simulink model "MPG_MG_PLL_orig"  (R2021b)
settings: Solver=VariableStepAuto  StartTime=0.0  StopTime=1  RelTol=1e-3
model workspace (MAT data in the model file):
  Ts = Simulink.Parameter
  Ts.Value = 5e-06
  Ts.DataType = 'auto'
  Ts.Complexity = 'real'
  Ts.Dimensions = [1 1]
  secondary_on = Simulink.Parameter
  secondary_on.DataType = 'auto'
  secondary_on.Complexity = 'real'
  secondary_on.Dimensions = [0 0]
values from neighbouring files (symbols this model uses):
  A = zeros(4,4)    [MPC_MG_script_raw_dmpc.m]    (also in MPG_MG_July.m = [0 1 1 1; 1 0 0 0; 1 0 0 0; 1 0 0 0]; MPG_MG_freq_script.m = ones(4) - eye(4); Script.m = [0 1 1 1 ; 1 0 1 1 ; 1 1 0 1 ; 1 1 1 0])
  C_f = 50e-6    (= 5e-05)    [Four_DG_MG_PrimaryOnlyScript.m]    (also in MPC_MG_script.m; MPC_MG_script_raw_dmpc.m; MPC_MG_secondary_script.m; MPG_MG_July.m)
  f_c = 5000    [Four_DG_MG_PrimaryOnlyScript.m]    (also in MPC_MG_script.m = 40000; MPC_MG_script_raw_dmpc.m = 40000; MPC_MG_secondary_script.m = 40000; MPG_MG_July.m = 50000)
  kL = 1e-5    (= 1e-05)    [Four_DG_MG_PrimaryOnlyScript.m]    (also in MPC_MG_script.m = 1e-08; MPC_MG_script_raw_dmpc.m = 1e-08; MPC_MG_secondary_script.m = 1e-07; MPG_MG_July.m = 1e-07)
  L_f = 1.35e-3    (= 0.00135)    [Four_DG_MG_PrimaryOnlyScript.m]    (also in MPC_MG_script.m; MPC_MG_script_raw_dmpc.m; MPC_MG_secondary_script.m; MPG_MG_July.m)
  L_in1 = 0.35e-3    (= 0.00035)    [Four_DG_MG_PrimaryOnlyScript.m]    (also in MPC_MG_script.m; MPC_MG_script_raw_dmpc.m; MPC_MG_secondary_script.m; MPG_MG_July.m)
  L_in2 = 0.35e-3    (= 0.00035)    [Four_DG_MG_PrimaryOnlyScript.m]    (also in MPC_MG_script.m; MPC_MG_script_raw_dmpc.m; MPC_MG_secondary_script.m; MPG_MG_July.m)
  L_in4 = 0.35e-3    (= 0.00035)    [Four_DG_MG_PrimaryOnlyScript.m]    (also in MPC_MG_script.m; MPC_MG_script_raw_dmpc.m; MPC_MG_secondary_script.m; MPG_MG_July.m)
  lambda1 = [30000 50000 90000 50000]'    [MPC_MG_script_raw_dmpc.m]    (also in MPG_MG_July.m = [4 4 4 4]'; MPG_MG_freq_script.m = [3 3 3 3]'; Script.m = [1 1 1 1]')
  lambda2 = [5 6 7 6]'    [MPC_MG_script_raw_dmpc.m]    (also in MPG_MG_July.m = [0.5e-2 0.5e-2 0.5e-2 0.5e-2]'; MPG_MG_freq_script.m = [1.1 1.9 1.5 1.2]'; Script.m = [0.8e-2 0.8e-2 0.8e-2 0.8e-2]')
  lambda3 = [80000 80000 900000 80000]'    [MPC_MG_script_raw_dmpc.m]    (also in MPG_MG_July.m = [1e-3 1e-3 1e-3 1e-3]'; MPG_MG_freq_script.m = [9e-4 1.2e-2 3e-3 3e-3]'; Script.m = [1.5e-3 1.5e-3 1.5e-3 1.5e-3]')
  LD_ref1 = 800e-6    (= 0.0008)    [Four_DG_MG_PrimaryOnlyScript.m]    (also in MPC_MG_script.m = 0.0003; MPC_MG_script_raw_dmpc.m = 0.0003; MPC_MG_secondary_script.m = 0.0001; MPG_MG_July.m = 0.0004)
  lo_co = 0.2    [Four_DG_MG_PrimaryOnlyScript.m]    (also in MPC_MG_script.m = 0.05; MPC_MG_script_raw_dmpc.m; MPC_MG_secondary_script.m = 0.08; MPG_MG_July.m = 0.15)
  m_p1 = 9.4e-5/droopDivide    (= 9.4e-05)    [Four_DG_MG_PrimaryOnlyScript.m]    (also in MPC_MG_script.m; MPC_MG_script_raw_dmpc.m; MPC_MG_secondary_script.m; MPG_MG_July.m)
  m_p2 = 9.4e-5/droopDivide    (= 9.4e-05)    [Four_DG_MG_PrimaryOnlyScript.m]    (also in MPC_MG_script.m; MPC_MG_script_raw_dmpc.m; MPC_MG_secondary_script.m; MPG_MG_July.m)
  m_p3 = 12.5e-5/droopDivide    (= 0.000125)    [Four_DG_MG_PrimaryOnlyScript.m]    (also in MPC_MG_script.m; MPC_MG_script_raw_dmpc.m; MPC_MG_secondary_script.m; MPG_MG_July.m)
  m_p4 = 12.5e-5/droopDivide    (= 0.000125)    [Four_DG_MG_PrimaryOnlyScript.m]    (also in MPC_MG_script.m; MPC_MG_script_raw_dmpc.m; MPC_MG_secondary_script.m; MPG_MG_July.m)
  N = 3    [MPG_MG_July.m]    (also in MPG_MG_freq_script.m = 2; Script.m = 5)
  n_q1 = 1.3e-3/droopDivide2    (= 0.00013)    [Four_DG_MG_PrimaryOnlyScript.m]    (also in MPC_MG_script.m; MPC_MG_script_raw_dmpc.m; MPC_MG_secondary_script.m; MPG_MG_July.m)
  n_q2 = 1.3e-3/droopDivide2    (= 0.00013)    [Four_DG_MG_PrimaryOnlyScript.m]    (also in MPC_MG_script.m; MPC_MG_script_raw_dmpc.m; MPC_MG_secondary_script.m; MPG_MG_July.m)
  n_q4 = 1.5e-3/droopDivide2    (= 0.00015)    [Four_DG_MG_PrimaryOnlyScript.m]    (also in MPC_MG_script.m; MPC_MG_script_raw_dmpc.m; MPC_MG_secondary_script.m; MPG_MG_July.m)
  Pmax = [45e3 45e3 37e3 37e3]'    [MPG_MG_July.m]    (also in MPG_MG_freq_script.m; Script.m)
  R_f = 0.1    [Four_DG_MG_PrimaryOnlyScript.m]    (also in MPC_MG_script.m; MPC_MG_script_raw_dmpc.m; MPC_MG_secondary_script.m; MPG_MG_July.m)
  R_in1 = 0.03    [Four_DG_MG_PrimaryOnlyScript.m]    (also in MPC_MG_script.m; MPC_MG_script_raw_dmpc.m; MPC_MG_secondary_script.m; MPG_MG_July.m)
  R_in2 = 0.03    [Four_DG_MG_PrimaryOnlyScript.m]    (also in MPC_MG_script.m; MPC_MG_script_raw_dmpc.m; MPC_MG_secondary_script.m; MPG_MG_July.m)
  R_in4 = 0.03    [Four_DG_MG_PrimaryOnlyScript.m]    (also in MPC_MG_script.m; MPC_MG_script_raw_dmpc.m; MPC_MG_secondary_script.m; MPG_MG_July.m)
  time_thresh = 0.6    [Four_DG_MG_PrimaryOnlyScript.m]    (also in MPC_MG_script_raw_dmpc.m = 1.5; MPC_MG_secondary_script.m = 2; MPG_MG_July.m = 0.5; MPG_MG_freq_script.m = 0.5)
  Ts = 10e-6    (= 1e-05)    [Four_DG_MG_PrimaryOnlyScript.m]    (also in MPC_MG_script.m; MPC_MG_script_raw_dmpc.m; MPC_MG_secondary_script.m; MPG_MG_July.m)
  Tsamp = 0.1    [MPG_MG_July.m]    (also in MPG_MG_freq_script.m; Script.m)
  V_nom = 220*sqrt(2)    [Four_DG_MG_PrimaryOnlyScript.m]    (also in MPC_MG_script.m; MPC_MG_script_raw_dmpc.m; MPC_MG_secondary_script.m; MPG_MG_July.m)
  Vdc = 600    [Four_DG_MG_PrimaryOnlyScript.m]    (also in MPC_MG_script.m; MPC_MG_script_raw_dmpc.m; MPC_MG_secondary_script.m; MPG_MG_July.m)
  w_c_high = 2*pi*50    (= 314.159265359)    [Four_DG_MG_PrimaryOnlyScript.m]    (also in MPC_MG_script.m; MPC_MG_script_raw_dmpc.m; MPC_MG_secondary_script.m; MPG_MG_July.m)
  w_nom = 2*pi*50    (= 314.159265359)    [Four_DG_MG_PrimaryOnlyScript.m]    (also in MPC_MG_script.m; MPC_MG_script_raw_dmpc.m; MPC_MG_secondary_script.m; MPG_MG_July.m)
undefined symbols (not defined in the file or in its folder): i
libraries: spsThreePhaseSeriesRLCBranchLib x18, spsabctodq0Lib x16, spsThreePhaseVIMeasurementLib x15, eeGeneralControl x15, dspswit3 x5, spsDCVoltageSourceLib x5, spsSeriesRLCBranchLib x5, spsTwoLevelConverterLib x5, slpidlib x5, spsAlphaBetaZerotodq0Lib x4, spsSecondOrderFilterLib x4, spsThreePhaseSeriesRLCLoadLib x2
(part 1 of 6)
settings Model: SimulationMode=accelerator  Creator=Linh  LastModifiedBy=Linh
settings SolverCC: AlgebraicLoopSolver=TrustRegion
settings DataIOCC: ReturnWorkspaceOutputs=off
settings DebuggingCC: SFMachineParentedDataDiag=warning

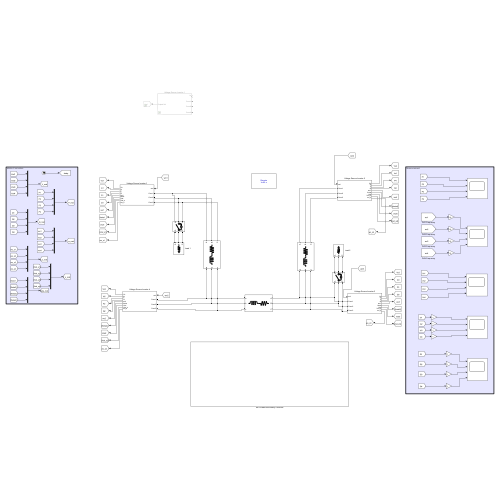
[thumbnail: Simulink's stored preview of the top-level diagram]
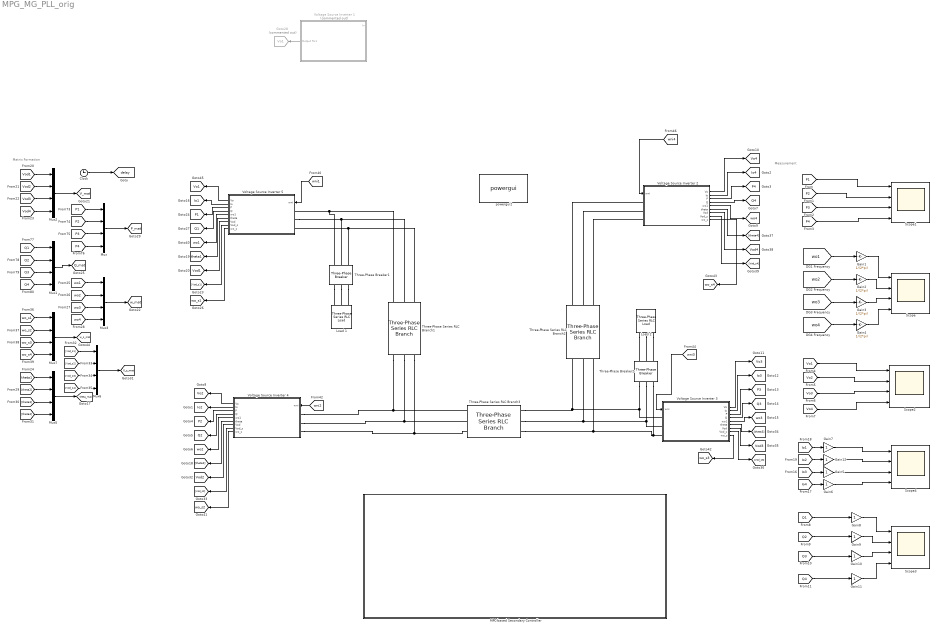
== system MPG_MG_PLL_orig ==
  note: Matrix Formation
  note: Measurement
  Clock : Clock
  Gain{1..4} (4 alike) : Gain  Gain=1/(2*pi)
  Gain{5..12} (8 alike) : Gain
  Goto28 : Goto  Commented=on  GotoTag=Vo1  TagVisibility=global
  Load 1 : spsThreePhaseSeriesRLCLoadLib/Three-Phase Series RLC Load  LConnTagsString=A|B|C  Configuration=Y (grounded)  NominalVoltage=220*sqrt(3)  Vabc=[1e3 1e3 1e3]  Vabcp=[1e3 1e3 1e3]  NominalFrequency=50  UnbalancedPower=off  ActivePower=4.285e3  InductivePower=0  CapacitivePower=0  Pabc=[10e3 9e3 11e3]  QLabc=[100 90 110]  QCabc=[100 90 110]  Pabcp=[10e3 9e3 11e3]  QLabcp=[100 90 110]  QCabcp=[100 90 110]  Measurements=Branch voltages and currents  LoadType=constant Z
  Load 2 : spsThreePhaseSeriesRLCLoadLib/Three-Phase Series RLC Load  LConnTagsString=A|B|C  Configuration=Y (grounded)  NominalVoltage=220*sqrt(3)  Vabc=[1e3 1e3 1e3]  Vabcp=[1e3 1e3 1e3]  NominalFrequency=50  UnbalancedPower=off  ActivePower=2.045e3  InductivePower=0  CapacitivePower=0  Pabc=[10e3 9e3 11e3]  QLabc=[100 90 110]  QCabc=[100 90 110]  Pabcp=[10e3 9e3 11e3]  QLabcp=[100 90 110]  QCabcp=[100 90 110]  Measurements=Branch voltages and currents  LoadType=constant Z
  MPC-based Secondary Controller : Subsystem
  Mux{,1..3,5..7} (7 alike) : Mux
  Scope{,1..4} (5 alike) : Scope  NumInputPorts=4
  Three-Phase Series RLC Branch1 : spsThreePhaseSeriesRLCBranchLib/Three-Phase Series RLC Branch  LConnTagsString=A|B|C  RConnTagsString=A|B|C  BranchType=RL  Resistance=0.01  Inductance=2.5e-3  Capacitance=1e-6  Measurements=Branch voltages and currents
  Three-Phase Series RLC Branch2 : spsThreePhaseSeriesRLCBranchLib/Three-Phase Series RLC Branch  LConnTagsString=A|B|C  RConnTagsString=A|B|C  BranchType=RL  Resistance=0.01  Inductance=2.5e-3  Capacitance=1e-6  Measurements=Branch voltages and currents
  Three-Phase Series RLC Branch3 : spsThreePhaseSeriesRLCBranchLib/Three-Phase Series RLC Branch  LConnTagsString=A|B|C  RConnTagsString=A|B|C  BranchType=RL  Resistance=0.01  Inductance=2.5e-3  Capacitance=1e-6  Measurements=Branch voltages and currents
  Three-Phase Breaker1 : spsThreePhaseBreakerLib/Three-Phase Breaker  InitialState=open  SwitchA=on  SwitchB=on  SwitchC=on  SwitchTimes=[0 11]  External=off  BreakerResistance=0.01  SnubberResistance=1e6  SnubberCapacitance=inf  Measurements=None
  Three-Phase Breaker2 : spsThreePhaseBreakerLib/Three-Phase Breaker  InitialState=open  SwitchA=on  SwitchB=on  SwitchC=on  SwitchTimes=[0.75 11]  External=off  BreakerResistance=0.01  SnubberResistance=1e6  SnubberCapacitance=inf  Measurements=None
  Voltage Source Inverter 1 : Subsystem  Commented=on  mask{w_nom=w_nom, V_nom=V_nom, modT=1/f_c, m_p=m_p2, n_q=n_q2, LD_ref=LD_ref1, k_LD=kL, w_c_high=[1 w_c_high], R_f=R_f, L_f=L_f, C_f=C_f, R_in=R_in2, L_in=L_in2}
      mask prompts: w_nom "Nominal frequency (radian)"; V_nom "Nominal voltage"; modT "Sampling Time"; m_p "P-w gain"; n_q "Q-V gain"; LD_ref "Reference virtual impedance (H)"; k_LD "Virtual impedance Q gain"; w_c_high "High-pass filter denominator:"; R_f "Inductor resistance:"; L_f "Filter inductance"; C_f "Filter capacitance"; R_in "Resistance coupling"; L_in "Inductance coupling"
      mask TypeOptions w_nom: w_nom/Value
      mask TypeOptions V_nom: V_nom/Value
      mask TypeOptions modT:
      | Model Predictive Control
      | /Ts
      mask TypeOptions m_p: Droop for secondary control2/Gain5/Gain
      mask TypeOptions n_q: Droop for secondary control2/Gain4/Gain
      mask TypeOptions LD_ref: LD_ref/Value
      mask TypeOptions k_LD: k_LD/Gain
      mask TypeOptions w_c_high: High-Pass Filter/Denominator
      mask TypeOptions R_f:
      | Three-Phase
      | Series RLC Branch/Resistance
      mask TypeOptions L_f:
      | Three-Phase
      | Series RLC Branch/Inductance
      mask TypeOptions C_f:
      | Three-Phase
      | Series RLC Branch2/Capacitance
      mask TypeOptions R_in:
      | Three-Phase
      | Series RLC Branch1/Resistance
      mask TypeOptions L_in:
      | Three-Phase
      | Series RLC Branch1/Inductance
      mask DialogControl ParameterGroupVar Prompt: Microgrid-wide values
      mask DialogControl Container5 Prompt: Droop value
      mask DialogControl Container8 Prompt: Filter
  Voltage Source Inverter 2 : Subsystem  mask{w_nom=w_nom, V_nom=V_nom, modT=1/f_c, m_p=m_p4, n_q=n_q4, LD_ref=LD_ref1, k_LD=kL, w_c_high=[1 w_c_high], R_f=R_f, L_f=L_f, C_f=C_f, R_in=R_in4, L_in=L_in4}
      mask prompts: w_nom "Nominal frequency (radian)"; V_nom "Nominal voltage"; modT "Sampling Time"; m_p "P-w gain"; n_q "Q-V gain"; LD_ref "Reference virtual impedance (H)"; k_LD "Virtual impedance Q gain"; w_c_high "High-pass filter denominator:"; R_f "Inductor resistance:"; L_f "Filter inductance"; C_f "Filter capacitance"; R_in "Resistance coupling"; L_in "Inductance coupling"
      mask TypeOptions w_nom: w_nom/Value
      mask TypeOptions V_nom: V_nom/Value
      mask TypeOptions modT:
      | Model Predictive Control
      | /Ts
      mask TypeOptions m_p: Droop for secondary control2/Gain5/Gain
      mask TypeOptions n_q: Droop for secondary control2/Gain4/Gain
      mask TypeOptions LD_ref: LD_ref/Value
      mask TypeOptions k_LD: k_LD/Gain
      mask TypeOptions w_c_high: High-Pass Filter/Denominator
      mask TypeOptions R_f:
      | Three-Phase
      | Series RLC Branch/Resistance
      mask TypeOptions L_f:
      | Three-Phase
      | Series RLC Branch/Inductance
      mask TypeOptions C_f:
      | Three-Phase
      | Series RLC Branch2/Capacitance
      mask TypeOptions R_in:
      | Three-Phase
      | Series RLC Branch1/Resistance
      mask TypeOptions L_in:
      | Three-Phase
      | Series RLC Branch1/Inductance
      mask DialogControl ParameterGroupVar Prompt: Microgrid-wide values
      mask DialogControl Container5 Prompt: Droop value
      mask DialogControl Container8 Prompt: Filter
  Voltage Source Inverter 3 : Subsystem  mask{w_nom=w_nom, V_nom=V_nom, modT=1/f_c, m_p=m_p4, n_q=n_q4, LD_ref=LD_ref1, k_LD=kL, w_c_high=[1 w_c_high], R_f=R_f, L_f=L_f, C_f=C_f, R_in=R_in4, L_in=L_in4}
      mask prompts: w_nom "Nominal frequency (radian)"; V_nom "Nominal voltage"; modT "Sampling Time"; m_p "P-w gain"; n_q "Q-V gain"; LD_ref "Reference virtual impedance (H)"; k_LD "Virtual impedance Q gain"; w_c_high "High-pass filter denominator:"; R_f "Inductor resistance:"; L_f "Filter inductance"; C_f "Filter capacitance"; R_in "Resistance coupling"; L_in "Inductance coupling"
      mask TypeOptions w_nom: w_nom/Value
      mask TypeOptions V_nom: V_nom/Value
      mask TypeOptions modT:
      | Model Predictive Control
      | /Ts
      mask TypeOptions m_p: Droop for secondary control2/Gain5/Gain
      mask TypeOptions n_q: Droop for secondary control2/Gain4/Gain
      mask TypeOptions LD_ref: LD_ref/Value
      mask TypeOptions k_LD: k_LD/Gain
      mask TypeOptions w_c_high: High-Pass Filter/Denominator
      mask TypeOptions R_f:
      | Three-Phase
      | Series RLC Branch/Resistance
      mask TypeOptions L_f:
      | Three-Phase
      | Series RLC Branch/Inductance
      mask TypeOptions C_f:
      | Three-Phase
      | Series RLC Branch2/Capacitance
      mask TypeOptions R_in:
      | Three-Phase
      | Series RLC Branch1/Resistance
      mask TypeOptions L_in:
      | Three-Phase
      | Series RLC Branch1/Inductance
      mask DialogControl ParameterGroupVar Prompt: Microgrid-wide values
      mask DialogControl Container5 Prompt: Droop value
      mask DialogControl Container8 Prompt: Filter
  Voltage Source Inverter 4 : Subsystem  mask{w_nom=w_nom, V_nom=V_nom, modT=1/f_c, m_p=m_p2, n_q=n_q2, LD_ref=LD_ref1, k_LD=kL, w_c_high=[1 w_c_high], R_f=R_f, L_f=L_f, C_f=C_f, R_in=R_in2, L_in=L_in2}
      mask prompts: w_nom "Nominal frequency (radian)"; V_nom "Nominal voltage"; modT "Sampling Time"; m_p "P-w gain"; n_q "Q-V gain"; LD_ref "Reference virtual impedance (H)"; k_LD "Virtual impedance Q gain"; w_c_high "High-pass filter denominator:"; R_f "Inductor resistance:"; L_f "Filter inductance"; C_f "Filter capacitance"; R_in "Resistance coupling"; L_in "Inductance coupling"
      mask TypeOptions w_nom: w_nom/Value
      mask TypeOptions V_nom: V_nom/Value
      mask TypeOptions modT:
      | Model Predictive Control
      | /Ts
      mask TypeOptions m_p: Droop for secondary control2/Gain5/Gain
      mask TypeOptions n_q: Droop for secondary control2/Gain4/Gain
      mask TypeOptions LD_ref: LD_ref/Value
      mask TypeOptions k_LD: k_LD/Gain
      mask TypeOptions w_c_high: High-Pass Filter/Denominator
      mask TypeOptions R_f:
      | Three-Phase
      | Series RLC Branch/Resistance
      mask TypeOptions L_f:
      | Three-Phase
      | Series RLC Branch/Inductance
      mask TypeOptions C_f:
      | Three-Phase
      | Series RLC Branch2/Capacitance
      mask TypeOptions R_in:
      | Three-Phase
      | Series RLC Branch1/Resistance
      mask TypeOptions L_in:
      | Three-Phase
      | Series RLC Branch1/Inductance
      mask DialogControl ParameterGroupVar Prompt: Microgrid-wide values
      mask DialogControl Container5 Prompt: Droop value
      mask DialogControl Container8 Prompt: Filter
  Voltage Source Inverter 5 : Subsystem  mask{w_nom=w_nom, V_nom=V_nom, modT=1/f_c, m_p=m_p1, n_q=n_q1, LD_ref=LD_ref1, k_LD=kL, w_c_high=[1 w_c_high], R_f=R_f, L_f=L_f, C_f=C_f, R_in=R_in1, L_in=L_in1}
      mask prompts: w_nom "Nominal frequency (radian)"; V_nom "Nominal voltage"; modT "Sampling Time"; m_p "P-w gain"; n_q "Q-V gain"; LD_ref "Reference virtual impedance (H)"; k_LD "Virtual impedance Q gain"; w_c_high "High-pass filter denominator:"; R_f "Inductor resistance:"; L_f "Filter inductance"; C_f "Filter capacitance"; R_in "Resistance coupling"; L_in "Inductance coupling"
      mask TypeOptions w_nom: w_nom/Value
      mask TypeOptions V_nom: V_nom/Value
      mask TypeOptions modT:
      | Model Predictive Control
      | /Ts
      mask TypeOptions m_p: Droop for secondary control2/Gain5/Gain
      mask TypeOptions n_q: Droop for secondary control2/Gain4/Gain
      mask TypeOptions LD_ref: LD_ref/Value
      mask TypeOptions k_LD: k_LD/Gain
      mask TypeOptions w_c_high: High-Pass Filter/Denominator
      mask TypeOptions R_f:
      | Three-Phase
      | Series RLC Branch/Resistance
      mask TypeOptions L_f:
      | Three-Phase
      | Series RLC Branch/Inductance
      mask TypeOptions C_f:
      | Three-Phase
      | Series RLC Branch2/Capacitance
      mask TypeOptions R_in:
      | Three-Phase
      | Series RLC Branch1/Resistance
      mask TypeOptions L_in:
      | Three-Phase
      | Series RLC Branch1/Inductance
      mask DialogControl ParameterGroupVar Prompt: Microgrid-wide values
      mask DialogControl Container5 Prompt: Droop value
      mask DialogControl Container8 Prompt: Filter
  powergui2 : spspowerguiLib/powergui  Priority=1  SimulationMode=Discrete  SampleTime=10e-6  frequency=60  Iterations=50  frequencyindice=0  Pbase=100e6  ErrMax=1e-4  UnitsV=kV  UnitsW=MW  buscounter=0  FunctionMessages=off  echomessages=off  EnableUseOfTLC=off  CurrentSourceSwitches=off  DisableSnubberDevices=off  DisableRonSwitches=off  DisableVfSwitches=off  DisplayEquations=off  AutomaticDiscreteSolvers=off  SolverType=Tustin/Backward Euler (TBE)  Interpol=off  ExternalGateDelay=off  methode=off  Ts=100  x0status=blocks  SPID=on  SwTol=0  HookPort=off  NonlinearTolerance=1e-4  nMaxIteration=100  ContinueOnMaxIteration=off  RestoreLinks=warning  ResistiveCurrentMeasurement=off  Frange=[0:2:500]  Ylog=off  Xlog=on  ShowGrid=off  save=off  variable=ZData  structure=ScopeData3  ZoomFFT=off  StartTime=0.5  cycles=1  DisplayStyle=1  fundamental=50  FreqAxis=off  MaxFrequency=1000  frequencyindicesteady=1  RmsSteady=1  display=off
  tag scope: Io1=global, Io2=global, Io3=global, Io4=global, P1=global, P2=global, P3=global, P4=global, P_mat=global, Q1=global, Q2=global, Q3=global, Q4=global, Q_mat=global, V_mat=global, V_s_mat=global, Vo1=global, Vo2=global, Vo3=global, Vo4=global, Vod1=global, Vod2=global, Vod3=global, Vod4=global, delay=global, theta1=global, theta_mat=global, w_mat=global, w_s_mat=global, wo1=global, wo2=global, wo3=global, wo4=global, wo_s1=global, wo_s2=global, wo_s3=global, wo_s4=global
  wires:
  Gain8/1 -> Scope3/1
  Gain11/1 -> Scope3/4
  [Q4] -> Gain11/1
  [Q1] -> Gain8/1
  [wo3] -> Gain3/1
  Gain2/1 -> Scope/2
  Gain4/1 -> Scope/4
  [wo1] -> Gain1/1
  [P1] -> Scope1/1
  [Vo4] -> Scope2/4
  [P3] -> Scope1/3
  [Q2] -> Gain9/1
  Gain9/1 -> Scope3/2
  [P2] -> Scope1/2
  Gain3/1 -> Scope/3
  [Vo2] -> Scope2/2
  [Vo3] -> Scope2/3
  [Vo1] -> Scope2/1
  [wo2] -> Gain2/1
  [Q3] -> Gain10/1
  Gain1/1 -> Scope/1
  [P4] -> Scope1/4
  Gain10/1 -> Scope3/3
  [wo4] -> Gain4/1
  [Io3] -> Gain5/1
  [Io1] -> Gain7/1
  [Io2] -> Gain12/1
  Gain6/1 -> Scope4/4
  [Io4] -> Gain6/1
  Gain5/1 -> Scope4/3
  Gain7/1 -> Scope4/1
  Gain12/1 -> Scope4/2
  Clock/1 -> [delay]
  [P1] -> Mux/1
  [P2] -> Mux/2
  [P3] -> Mux/3
  [P4] -> Mux/4
  Mux/1 -> [P_mat]
  [Q3] -> Mux1/3
  [Q4] -> Mux1/4
  [Q1] -> Mux1/1
  Mux1/1 -> [Q_mat]
  [Q2] -> Mux1/2
  [Vod3] -> Mux2/3
  [Vod4] -> Mux2/4
  [Vod1] -> Mux2/1
  Mux2/1 -> [V_mat]
  [Vod2] -> Mux2/2
  [wo3] -> Mux3/3
  [wo4] -> Mux3/4
  [wo1] -> Mux3/1
  Mux3/1 -> [w_mat]
  [wo2] -> Mux3/2
  Voltage Source Inverter 2/1(Vo) -> [Vo4]
  Voltage Source Inverter 2/2(Io) -> [Io4]
  Voltage Source Inverter 2/4(Q) -> [Q4]
  Voltage Source Inverter 2/3(P) -> [P4]
  Voltage Source Inverter 2/5(wo1) -> [wo4]
  Voltage Source Inverter 3/5(wo1) -> [wo3]
  Voltage Source Inverter 3/4(Q) -> [Q3]
  Voltage Source Inverter 3/1(Vo) -> [Vo3]
  Voltage Source Inverter 3/3(P) -> [P3]
  Voltage Source Inverter 3/2(Io) -> [Io3]
  [theta1] -> Mux5/1
  [theta3] -> Mux5/3
  [theta2] -> Mux5/2
  Mux5/1 -> [theta_mat]
  [theta4] -> Mux5/4
  [Vod_s2] -> Mux6/2
  [Vod_s3] -> Mux6/3
  [Vod_s1] -> Mux6/1
  Mux6/1 -> [V_s_mat]
  [Vod_s4] -> Mux6/4
  Voltage Source Inverter 4/1(Vo) -> [Vo2]
  Voltage Source Inverter 4/2(Io) -> [Io2]
  Voltage Source Inverter 4/3(P) -> [P2]
  Voltage Source Inverter 4/4(Q) -> [Q2]
  Voltage Source Inverter 4/5(wo1) -> [wo2]
  Voltage Source Inverter 4/6(theta) -> [theta2]
  Voltage Source Inverter 4/7(Vod) -> [Vod2]
  Voltage Source Inverter 4/8(Vod_s) -> [Vod_s2]
  Voltage Source Inverter 3/6(theta) -> [theta3]
  Voltage Source Inverter 3/7(Vod) -> [Vod3]
  Voltage Source Inverter 3/8(Vod_s) -> [Vod_s3]
  Voltage Source Inverter 2/6(theta) -> [theta4]
  Voltage Source Inverter 2/7(Vod) -> [Vod4]
  Voltage Source Inverter 2/8(Vod_s) -> [Vod_s4]
  Voltage Source Inverter 4/9(wo_s) -> [wo_s2]
  Voltage Source Inverter 3/9(wo_s) -> [wo_s3]
  Voltage Source Inverter 2/9(wo_s) -> [wo_s4]
  [wo_s3] -> Mux7/3
  [wo_s2] -> Mux7/2
  [wo_s4] -> Mux7/4
  Mux7/1 -> [w_s_mat]
  [wo_s1] -> Mux7/1
  Voltage Source Inverter 1/1(Output 9x1) -> Goto28/1
  Voltage Source Inverter 5/4(Q) -> [Q1]
  Voltage Source Inverter 5/9(wo_s) -> [wo_s1]
  Voltage Source Inverter 5/3(P) -> [P1]
  Voltage Source Inverter 5/2(Io) -> [Io1]
  Voltage Source Inverter 5/5(wo1) -> [wo1]
  Voltage Source Inverter 5/6(theta) -> [theta1]
  Voltage Source Inverter 5/1(Vo) -> [Vo1]
  Voltage Source Inverter 5/7(Vod) -> [Vod1]
  Voltage Source Inverter 5/8(Vod_s) -> [Vod_s1]
  [wni1] -> Voltage Source Inverter 5/1(wni)
  [wni2] -> Voltage Source Inverter 4/1(wni)
  [wni3] -> Voltage Source Inverter 3/1(wni)
  [wni4] -> Voltage Source Inverter 2/1(wni)
  connections:
  Three-Phase Series RLC Branch1/RConn2 -- Voltage Source Inverter 4/LConn2 -- Three-Phase Series RLC Branch3/RConn2
  Voltage Source Inverter 4/LConn1 -- Three-Phase Series RLC Branch3/RConn1 -- Three-Phase Series RLC Branch1/RConn1
  Three-Phase Series RLC Branch1/RConn3 -- Voltage Source Inverter 4/LConn3 -- Three-Phase Series RLC Branch3/RConn3
  Three-Phase Series RLC Branch2/RConn2 -- Three-Phase Series RLC Branch3/LConn2 -- Three-Phase Breaker2/LConn2 -- Voltage Source Inverter 3/LConn2
  Three-Phase Series RLC Branch2/RConn1 -- Three-Phase Series RLC Branch3/LConn1 -- Voltage Source Inverter 3/LConn1 -- Three-Phase Breaker2/LConn1
  Three-Phase Series RLC Branch2/RConn3 -- Three-Phase Series RLC Branch3/LConn3 -- Three-Phase Breaker2/LConn3 -- Voltage Source Inverter 3/LConn3
  Voltage Source Inverter 5/LConn2 -- Three-Phase Series RLC Branch1/LConn2 -- Three-Phase Breaker1/RConn2
  Voltage Source Inverter 5/LConn1 -- Three-Phase Series RLC Branch1/LConn1 -- Three-Phase Breaker1/RConn1
  Voltage Source Inverter 5/LConn3 -- Three-Phase Series RLC Branch1/LConn3 -- Three-Phase Breaker1/RConn3
  Three-Phase Series RLC Branch2/LConn1 -- Voltage Source Inverter 2/LConn1
  Three-Phase Series RLC Branch2/LConn2 -- Voltage Source Inverter 2/LConn2
  Three-Phase Series RLC Branch2/LConn3 -- Voltage Source Inverter 2/LConn3
  Load 2/LConn1 -- Three-Phase Breaker2/RConn1
  Load 2/LConn2 -- Three-Phase Breaker2/RConn2
  Load 2/LConn3 -- Three-Phase Breaker2/RConn3
  Three-Phase Breaker1/LConn1 -- Load 1/LConn1
  Three-Phase Breaker1/LConn2 -- Load 1/LConn2
  Three-Phase Breaker1/LConn3 -- Load 1/LConn3

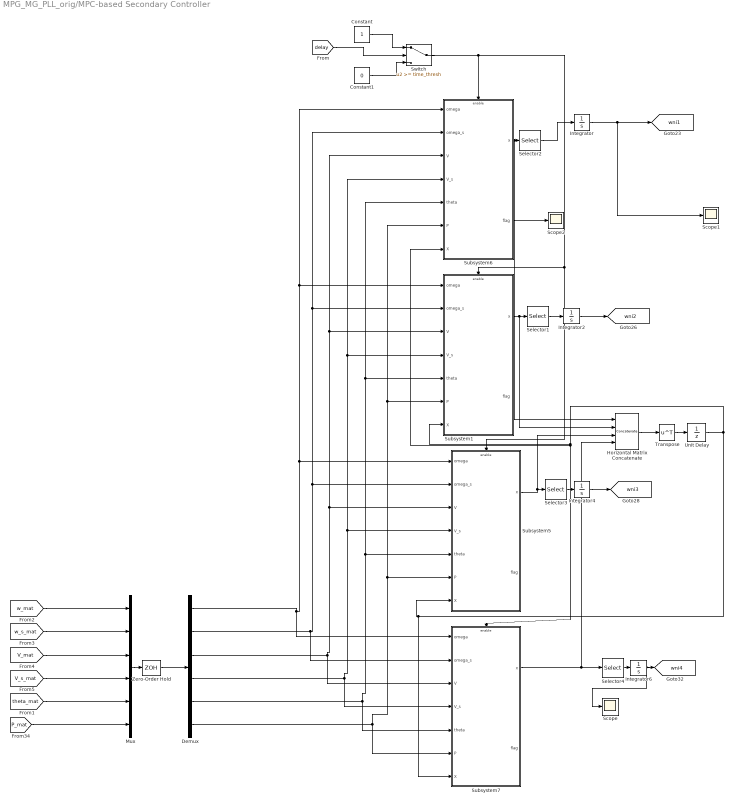
== system MPG_MG_PLL_orig/MPC-based Secondary Controller ==
  Constant : Constant
  Constant1 : Constant  Value=0
  Demux : Demux  Outputs=6
  Horizontal Matrix Concatenate : Concatenate  NumInputs=4  Mode=Multidimensional array  ConcatenateDimension=2
  Integrator{,2,4,6} (4 alike) : Integrator
  Mux : Mux  Inputs=6
  Scope : Scope
  Scope1 : Scope
  Scope2 : Scope
  Selector{1..4} (4 alike) : Selector  InputPortWidth=5*N  IndexOptions=Index vector (dialog)  Indices=[N+1]  OutputSizes=1
  Subsystem1 : Subsystem  mask{L_f=L_in1, a=2, Mpw=m_p2, Tsec=Tsamp, lambda1=lambda1, lambda2=lambda2, lambda3=lambda3, Pmax=Pmax, aij=A, N=N}
      mask prompts: L_f "Filter Inductor"; N "Horizon"
  Subsystem5 : Subsystem  mask{L_f=L_in1, a=3, Mpw=m_p3, Tsec=Tsamp, lambda1=lambda1, lambda2=lambda2, lambda3=lambda3, Pmax=Pmax, aij=A, N=N}
      mask prompts: L_f "Filter Inductor"; N "Horizon"
  Subsystem6 : Subsystem  mask{L_f=L_in1, a=1, Mpw=m_p4, Tsec=Tsamp, lambda1=lambda1, lambda2=lambda2, lambda3=lambda3, Pmax=Pmax, aij=A, N=N}
      mask prompts: L_f "Filter Inductor"; N "Horizon"
  Subsystem7 : Subsystem  mask{L_f=L_in1, a=4, Mpw=m_p4, Tsec=Tsamp, lambda1=lambda1, lambda2=lambda2, lambda3=lambda3, Pmax=Pmax, aij=A, N=N}
      mask prompts: L_f "Filter Inductor"; N "Horizon"
  Switch : Switch  Threshold=time_thresh
  Transpose : Math  Operator=transpose  SaturateOnIntegerOverflow=on
  Unit Delay : UnitDelay  SampleTime=Ts  HasFrameUpgradeWarning=on
  Zero-Order Hold : ZeroOrderHold  SampleTime=Tsamp
  tag scope: wni1=global, wni2=global, wni3=global, wni4=global
  wires:
  Integrator4/1 -> [wni3]
  Integrator/1 -> [wni1], Scope1/1
  Integrator2/1 -> [wni2]
  [w_s_mat] -> Mux/2
  [V_mat] -> Mux/3
  [V_s_mat] -> Mux/4
  [theta_mat] -> Mux/5
  [P_mat] -> Mux/6
  [w_mat] -> Mux/1
  [delay] -> Switch/2
  Constant/1 -> Switch/1
  Constant1/1 -> Switch/3
  Switch/1 -> Subsystem6/Enable, Subsystem5/Enable, Subsystem1/Enable
  Subsystem6/1(x) -> Selector2/1, Horizontal Matrix Concatenate/1
  Subsystem5/1(x) -> Selector3/1, Horizontal Matrix Concatenate/3
  Horizontal Matrix Concatenate/1 -> Transpose/1
  Transpose/1 -> Unit Delay/1
  Subsystem6/2(flag) -> Scope2/1
  Selector2/1 -> Integrator/1
  Subsystem1/1(x) -> Horizontal Matrix Concatenate/2, Selector1/1
  Selector1/1 -> Integrator2/1
  Selector3/1 -> Integrator4/1
  Subsystem7/1(x) -> Horizontal Matrix Concatenate/4, Selector4/1
  Selector4/1 -> Integrator6/1
  Demux/1 -> Subsystem7/1(omega), Subsystem5/1(omega), Subsystem6/1(omega), Subsystem1/1(omega)
  Demux/2 -> Subsystem7/2(omega_s), Subsystem6/2(omega_s), Subsystem1/2(omega_s), Subsystem5/2(omega_s)
  Demux/3 -> Subsystem6/3(V), Subsystem1/3(V), Subsystem5/3(V), Subsystem7/3(V)
  Demux/4 -> Subsystem7/4(V_s), Subsystem6/4(V_s), Subsystem1/4(V_s), Subsystem5/4(V_s)
  Demux/5 -> Subsystem6/5(theta), Subsystem1/5(theta), Subsystem5/5(theta), Subsystem7/5(theta)
  Demux/6 -> Subsystem6/6(P), Subsystem1/6(P), Subsystem5/6(P), Subsystem7/6(P)
  Integrator6/1 -> Scope/1, [wni4]
  Unit Delay/1 -> Subsystem7/7(X), Subsystem5/7(X), Subsystem6/7(X), Subsystem7/Enable, Subsystem1/7(X)
  Mux/1 -> Zero-Order Hold/1
  Zero-Order Hold/1 -> Demux/1

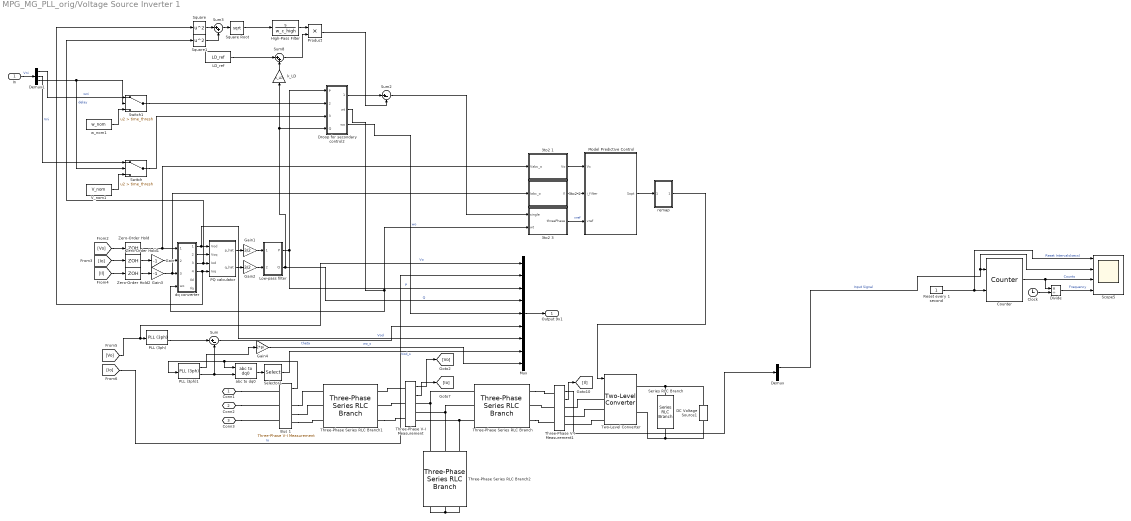
== system MPG_MG_PLL_orig/Voltage Source Inverter 1 ==
  In : Inport
  3to2 1 : Subsystem
  3to2 2 : Subsystem
  3to2 3 : Subsystem
  Bus 1 : spsThreePhaseVIMeasurementLib/Three-Phase V-I Measurement  VoltageMeasurement=phase-to-ground  SetLabelV=off  LabelV=Vbus  Vpu=off  VpuLL=off  CurrentMeasurement=yes  SetLabelI=off  LabelI=Ibus  Ipu=off  Pbase=100e6  Vbase=380  OutputType=Complex  PhasorSimulation=off  PSBequivalent=0
  Clock : Clock
  Counter : dspswit3/Counter  Direction=Up  CountEvent=Rising edge  CounterSize=User defined  MaxCount=5e5  InitialCount=0  Output=Count  HitValue=1  ResetInput=on  SamplesPerFrame=1  Ts=1  CntDtype=double  HitDtype=Logical
  DC Voltage Source1 : spsDCVoltageSourceLib/DC Voltage Source  Amplitude=Vdc  Measurements=None
  Demux : Demux  Outputs=3
  Demux1 : Demux  Outputs=3
  Divide : Product  Inputs=*/
  Droop for secondary control2 : Subsystem
  Gain : Gain  Gain=-1
  Gain1 : Gain  Gain=3/2
  Gain2 : Gain  Gain=3/2
  Gain3 : Gain  Gain=-1
  Gain4 : Gain  Gain=2*pi
  High-Pass Filter : TransferFcn  Numerator=[1 0]  Denominator=w_c_high
  LD_ref : Constant  Value=LD_ref
  Low-pass filter : Subsystem
  "Model Predictive Control " : MATLAB Function  TreatAsAtomicUnit=on  mask{Ts=modT, Cfilter=C_f, Lfilter=L_f, Vdc=Vdc}
      mask prompts: Ts "Sampling Time"; Cfilter "Filter Capacitor"; Lfilter "Filter Inductance"; Vdc "Input DC Voltage"
  Mux : Mux  Inputs=9
  PLL (3ph) : spsPLL3phLib/PLL (3ph)  Fmin=45  Par_Init=[0, 50]  ParK=[180, 3200, 1]  TcD=1e-3  MaxRateChangeFreq=12  FilterCutOffFreq=25  Ts=1e-3  AGC=on
  PLL (3ph)1 : spsPLL3phLib/PLL (3ph)  Fmin=45  Par_Init=[0, 50]  ParK=[180, 3200, 1]  TcD=1e-3  MaxRateChangeFreq=12  FilterCutOffFreq=25  Ts=1e-3  AGC=on
  PQ calculator : Subsystem
  Product : Product
  Reset every 1 second : Constant
  Scope5 : Scope  NumInputPorts=4
  Selector1 : Selector  InputPortWidth=3  IndexOptions=Index vector (dialog)  Indices=[1]  OutputSizes=1
  Series RLC Branch : spsSeriesRLCBranchLib/Series RLC Branch  LConnTagsString=__new0  RConnTagsString=__new0  BranchType=RC  Resistance=30  Inductance=1e-3  SetiL0=off  InitialCurrent=0  Capacitance=80e-6  Setx0=off  InitialVoltage=0  Measurements=None
  Square : Math  Operator=square  SaturateOnIntegerOverflow=on
  Square Root : Sqrt  SaturateOnIntegerOverflow=on
  Square1 : Math  Operator=square  SaturateOnIntegerOverflow=on
  Sum : Sum  Inputs=|+-
  Sum2 : Sum  Inputs=|+-
  Sum3 : Sum  Inputs=|++
  Sum8 : Sum  Inputs=|++
  Switch : Switch  Criteria=u2 > Threshold  Threshold=time_thresh
  Switch1 : Switch  Criteria=u2 > Threshold  Threshold=time_thresh
  Three-Phase Series RLC Branch : spsThreePhaseSeriesRLCBranchLib/Three-Phase Series RLC Branch  LConnTagsString=A|B|C  RConnTagsString=A|B|C  BranchType=RL  Resistance=R_f  Inductance=L_f  Capacitance=1e-6  Measurements=None
  Three-Phase Series RLC Branch1 : spsThreePhaseSeriesRLCBranchLib/Three-Phase Series RLC Branch  LConnTagsString=A|B|C  RConnTagsString=A|B|C  BranchType=RL  Resistance=R_in  Inductance=L_in  Capacitance=1e-6  Measurements=None
  Three-Phase Series RLC Branch2 : spsThreePhaseSeriesRLCBranchLib/Three-Phase Series RLC Branch  LConnTagsString=A|B|C  RConnTagsString=A|B|C  BranchType=C  Resistance=R_f  Inductance=1e-3  Capacitance=C_f  Measurements=None
  Three-Phase V-I Measurement : spsThreePhaseVIMeasurementLib/Three-Phase V-I Measurement  VoltageMeasurement=phase-to-ground  SetLabelV=off  LabelV=Vo1  Vpu=off  VpuLL=off  CurrentMeasurement=yes  SetLabelI=off  LabelI=Io1  Ipu=off  Pbase=100e6  Vbase=500e3  OutputType=Complex  PhasorSimulation=off  PSBequivalent=0
  Three-Phase V-I Measurement1 : spsThreePhaseVIMeasurementLib/Three-Phase V-I Measurement  VoltageMeasurement=phase-to-ground  SetLabelV=off  LabelV=Vl2  Vpu=off  VpuLL=off  CurrentMeasurement=yes  SetLabelI=off  LabelI=Il2  Ipu=off  Pbase=100e6  Vbase=500e3  OutputType=Complex  PhasorSimulation=off  PSBequivalent=0
  Two-Level Converter : spsTwoLevelConverterLib/Two-Level Converter  ModelType=Switching devices  Ron=1e-3  Rs=1e6  Cs=inf  Vforward=[0,0]  Ron_Diode=1e-3  Rs_Diode=1e6  Cs_Diode=inf  Vf_Diode=1e-3  Rs_CurrentSource=inf
      settings: SourceProductBaseCode=PS
  V_nom1 : Constant  Value=V_nom
  Zero-Order Hold : ZeroOrderHold  SampleTime=modT
  Zero-Order Hold1 : ZeroOrderHold  SampleTime=modT
  Zero-Order Hold2 : ZeroOrderHold  SampleTime=modT
  abc to dq0 : spsabctodq0Lib/abc to dq0  Alignment=90 degrees behind phase A axis
  dq converter : Subsystem
  k_LD : Gain  Gain=k_LD
  remap : Subsystem
  w_nom1 : Constant  Value=w_nom
  Conn1 : PMIOPort  Side=Left
  Conn2 : PMIOPort  Port=2  Side=Left
  Conn3 : PMIOPort  Port=3  Side=Left
  Output 9x1 : Outport
  wires:
  Gain/1 -> dq converter/2(Iodq)
  Droop for secondary control2/2(wt) -> dq converter/4(wo), 3to2 3/2("wt ")
  Gain2/1 -> Low-pass filter/2(q_hat)
  PQ calculator/2(q_hat) -> Gain2/1
  Gain1/1 -> Low-pass filter/1(p_hat)
  dq converter/2(Voq) -> PQ calculator/2(Voq)
  [Il] -> Zero-Order Hold2/1
  PQ calculator/1(p_hat) -> Gain1/1
  [Io] -> Zero-Order Hold1/1
  dq converter/1(Vod) -> Mux/7, PQ calculator/1(Vod)  "Vod"
  [Vo] -> Mux/1, PLL (3ph)/1  "Vo"
  [Io] -> Mux/2  "Io"
  Three-Phase V-I Measurement/1 -> [Vo]
  Three-Phase V-I Measurement/2 -> [Io]
  Three-Phase V-I Measurement1/2 -> [Il]
  3to2 1/1(Vo) -> "Model Predictive Control "/1(Vc)
  3to2 3/1(threePhase) -> "Model Predictive Control "/3(vref)  "vref"
  3to2 2/1(Il) -> "Model Predictive Control "/2(i_filter)
  [Vo] -> Zero-Order Hold/1
  "Model Predictive Control "/1(Sopt) -> remap/1(In1)
  Gain3/1 -> 3to2 2/1("Iabc_o "), dq converter/3(Ildq)
  remap/1(Out1) -> Two-Level Converter/1
  Zero-Order Hold/1 -> 3to2 1/1("Vabc_o "), dq converter/1(Vodq)
  Zero-Order Hold1/1 -> Gain/1
  Zero-Order Hold2/1 -> Gain3/1
  Sum2/1 -> 3to2 3/1("single ")
  Three-Phase V-I Measurement1/1 -> Demux/1
  Demux/1 -> Counter/1, Scope5/2  "Input Signal"
  Clock/1 -> Divide/2
  Reset every 1 second/1 -> Scope5/1, Counter/2  "Reset Intervals(secs)"
  Counter/1 -> Scope5/3, Divide/1  "Counts"
  Divide/1 -> Scope5/4  "Frequency"
  Square1/1 -> Sum3/2
  Sum3/1 -> Square Root/1
  Sum8/1 -> Product/2
  k_LD/1 -> Sum8/2
  Square Root/1 -> High-Pass Filter/1
  Low-pass filter/2(Q) -> Mux/4, k_LD/1, Droop for secondary control2/4(Q)  "Q"
  Droop for secondary control2/1(Vref) -> Sum2/1
  LD_ref/1 -> Sum8/1
  dq converter/3(Iod) -> Square1/1, PQ calculator/3(Iod)
  Droop for secondary control2/3(wo) -> Mux/5  "wo"
  Product/1 -> Sum2/2
  dq converter/4(Ioq) -> Square/1, PQ calculator/4(Ioq)
  High-Pass Filter/1 -> Product/1
  Low-pass filter/1(P) -> Droop for secondary control2/1(P), Mux/3  "P"
  Square/1 -> Sum3/1
  w_nom1/1 -> Switch1/3
  Demux1/3 -> Switch/2, Switch1/2  "delay"
  V_nom1/1 -> Switch/3
  Switch1/1 -> Droop for secondary control2/2(w_nom)
  Switch/1 -> Droop for secondary control2/3(V_nom)
  Bus 1/1 -> abc to dq0/1, PLL (3ph)1/1
  PLL (3ph)/2 -> Sum/1
  PLL (3ph)1/2 -> abc to dq0/2, Sum/2
  Sum/1 -> Mux/6  "theta"
  abc to dq0/1 -> Selector1/1
  Selector1/1 -> Mux/8  "Vod_s"
  PLL (3ph)1/1 -> Gain4/1
  Gain4/1 -> Mux/9  "wo_s"
  Mux/1 -> Output 9x1/1
  In/1 -> Demux1/1  "Vni"
  Demux1/1 -> Switch1/1  "wni"
  Demux1/2 -> Switch/1  "Vni"
  connections:
  Three-Phase Series RLC Branch2/LConn1 -- Three-Phase V-I Measurement/RConn1 -- Three-Phase Series RLC Branch/LConn1
  Two-Level Converter/RConn1 -- DC Voltage Source1/RConn1 -- Series RLC Branch/LConn1
  Three-Phase Series RLC Branch2/RConn3 -- Three-Phase Series RLC Branch2/RConn1 -- Three-Phase Series RLC Branch2/RConn2
  Three-Phase Series RLC Branch2/LConn3 -- Three-Phase Series RLC Branch/LConn3 -- Three-Phase V-I Measurement/RConn3
  Two-Level Converter/RConn2 -- Series RLC Branch/RConn1 -- DC Voltage Source1/LConn1
  Three-Phase Series RLC Branch/LConn2 -- Three-Phase V-I Measurement/RConn2 -- Three-Phase Series RLC Branch2/LConn2
  Two-Level Converter/LConn1 -- Three-Phase V-I Measurement1/RConn1
  Three-Phase V-I Measurement1/LConn2 -- Three-Phase Series RLC Branch/RConn2
  Two-Level Converter/LConn2 -- Three-Phase V-I Measurement1/RConn2
  Two-Level Converter/LConn3 -- Three-Phase V-I Measurement1/RConn3
  Three-Phase Series RLC Branch/RConn1 -- Three-Phase V-I Measurement1/LConn1
  Three-Phase V-I Measurement/LConn1 -- Three-Phase Series RLC Branch1/RConn1
  Three-Phase V-I Measurement/LConn2 -- Three-Phase Series RLC Branch1/RConn2
  Three-Phase Series RLC Branch1/RConn3 -- Three-Phase V-I Measurement/LConn3
  Three-Phase Series RLC Branch/RConn3 -- Three-Phase V-I Measurement1/LConn3
  Conn1/RConn1 -- Bus 1/LConn1
  Conn2/RConn1 -- Bus 1/LConn2
  Conn3/RConn1 -- Bus 1/LConn3
  Bus 1/RConn1 -- Three-Phase Series RLC Branch1/LConn1
  Bus 1/RConn2 -- Three-Phase Series RLC Branch1/LConn2
  Bus 1/RConn3 -- Three-Phase Series RLC Branch1/LConn3

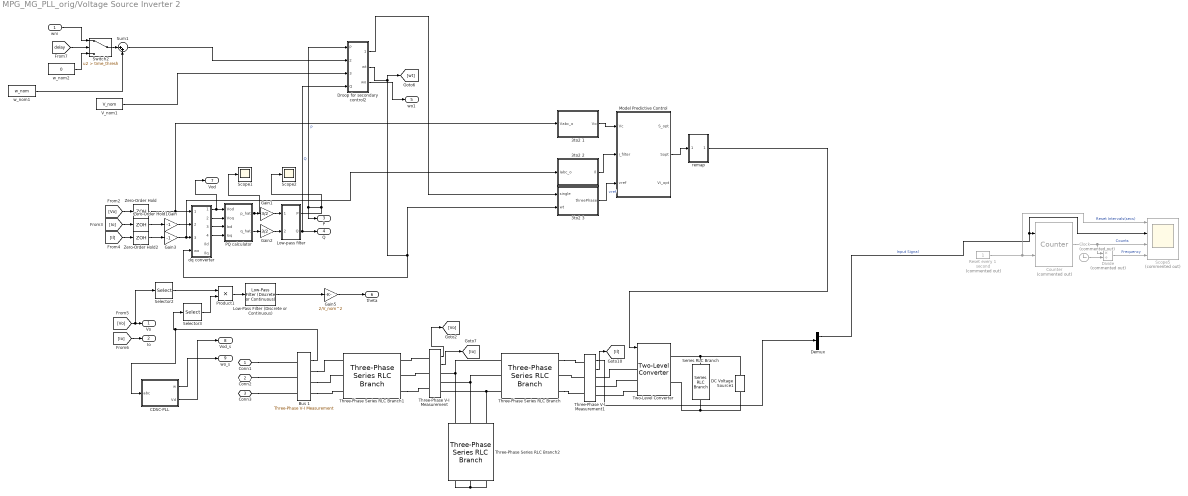
== system MPG_MG_PLL_orig/Voltage Source Inverter 2 ==
  wni : Inport
  3to2 1 : Subsystem
  3to2 2 : Subsystem
  3to2 3 : Subsystem
  Bus 1 : spsThreePhaseVIMeasurementLib/Three-Phase V-I Measurement  VoltageMeasurement=phase-to-ground  SetLabelV=off  LabelV=Vbus  Vpu=off  VpuLL=off  CurrentMeasurement=no  SetLabelI=off  LabelI=Ibus  Ipu=off  Pbase=100e6  Vbase=380  OutputType=Complex  PhasorSimulation=off  PSBequivalent=0
  CDSC-PLL : Subsystem  mask{hr=7}
      mask prompts: hr "Required Component Extraction (hr)"
  Clock : Clock  Commented=on
  Counter : dspswit3/Counter  Commented=on  Direction=Up  CountEvent=Rising edge  CounterSize=User defined  MaxCount=5e5  InitialCount=0  Output=Count  HitValue=1  ResetInput=on  SamplesPerFrame=1  Ts=1  CntDtype=double  HitDtype=Logical
  DC Voltage Source1 : spsDCVoltageSourceLib/DC Voltage Source  Amplitude=Vdc  Measurements=None
  Demux : Demux  Outputs=3
  Divide : Product  Commented=on  Inputs=*/
  Droop for secondary control2 : Subsystem
  Gain : Gain  Gain=-1
  Gain1 : Gain  Gain=3/2
  Gain2 : Gain  Gain=3/2
  Gain3 : Gain  Gain=-1
  Gain5 : Gain  Gain=2/V_nom^2
  Low-Pass Filter (Discrete or Continuous) : eeGeneralControl/Low-Pass Filter (Discrete or Continuous)  K=1  T=0.1  B=inf  A=-inf  init_option=Inherited from block input  x0=0  Ts=-1
  Low-pass filter : Subsystem
  "Model Predictive Control " : MATLAB Function  TreatAsAtomicUnit=on  mask{Ts=modT, Cfilter=C_f, Lfilter=L_f, Vdc=Vdc}
      mask prompts: Ts "Sampling Time"; Cfilter "Filter Capacitor"; Lfilter "Filter Inductance"; Vdc "Input DC Voltage"
  PQ calculator : Subsystem
  Product1 : Product
  Reset every 1 second : Constant  Commented=on
  Scope1 : Scope
  Scope2 : Scope
  Scope5 : Scope  Commented=on  NumInputPorts=4
  Selector2 : Selector  InputPortWidth=3  IndexOptions=Index vector (dialog)  Indices=[1]  OutputSizes=1
  Selector3 : Selector  InputPortWidth=3  IndexOptions=Index vector (dialog)  Indices=[1]  OutputSizes=1
  Series RLC Branch : spsSeriesRLCBranchLib/Series RLC Branch  LConnTagsString=__new0  RConnTagsString=__new0  BranchType=RC  Resistance=30  Inductance=1e-3  SetiL0=off  InitialCurrent=0  Capacitance=80e-6  Setx0=off  InitialVoltage=0  Measurements=None
  Sum1 : Sum  Inputs=|++
  Switch2 : Switch  Criteria=u2 > Threshold  Threshold=time_thresh
  Three-Phase Series RLC Branch : spsThreePhaseSeriesRLCBranchLib/Three-Phase Series RLC Branch  LConnTagsString=A|B|C  RConnTagsString=A|B|C  BranchType=RL  Resistance=R_f  Inductance=L_f  Capacitance=1e-6  Measurements=None
  Three-Phase Series RLC Branch1 : spsThreePhaseSeriesRLCBranchLib/Three-Phase Series RLC Branch  LConnTagsString=A|B|C  RConnTagsString=A|B|C  BranchType=RL  Resistance=R_in  Inductance=L_in  Capacitance=1e-6  Measurements=None
  Three-Phase Series RLC Branch2 : spsThreePhaseSeriesRLCBranchLib/Three-Phase Series RLC Branch  LConnTagsString=A|B|C  RConnTagsString=A|B|C  BranchType=C  Resistance=R_f  Inductance=1e-3  Capacitance=C_f  Measurements=None
  Three-Phase V-I Measurement : spsThreePhaseVIMeasurementLib/Three-Phase V-I Measurement  VoltageMeasurement=phase-to-ground  SetLabelV=off  LabelV=Vo1  Vpu=off  VpuLL=off  CurrentMeasurement=yes  SetLabelI=off  LabelI=Io1  Ipu=off  Pbase=100e6  Vbase=500e3  OutputType=Complex  PhasorSimulation=off  PSBequivalent=0
  Three-Phase V-I Measurement1 : spsThreePhaseVIMeasurementLib/Three-Phase V-I Measurement  VoltageMeasurement=phase-to-ground  SetLabelV=off  LabelV=Vl2  Vpu=off  VpuLL=off  CurrentMeasurement=yes  SetLabelI=off  LabelI=Il2  Ipu=off  Pbase=100e6  Vbase=500e3  OutputType=Complex  PhasorSimulation=off  PSBequivalent=0
  Two-Level Converter : spsTwoLevelConverterLib/Two-Level Converter  ModelType=Switching devices  Ron=1e-3  Rs=1e6  Cs=inf  Vforward=[0,0]  Ron_Diode=1e-3  Rs_Diode=1e6  Cs_Diode=inf  Vf_Diode=1e-3  Rs_CurrentSource=inf
      settings: SourceProductBaseCode=PS
  V_nom1 : Constant  Value=V_nom
  Zero-Order Hold : ZeroOrderHold  SampleTime=modT
  Zero-Order Hold1 : ZeroOrderHold  SampleTime=modT
  Zero-Order Hold2 : ZeroOrderHold  SampleTime=modT
  dq converter : Subsystem
  remap : Subsystem
  w_nom1 : Constant  Value=w_nom
  w_nom2 : Constant  Value=0
  Conn1 : PMIOPort  Side=Left
  Conn2 : PMIOPort  Port=2  Side=Left
  Conn3 : PMIOPort  Port=3  Side=Left
  Vo : Outport
  Io : Outport  Port=2
  P : Outport  Port=3
  Q : Outport  Port=4
  wo1 : Outport  Port=5
  theta : Outport  Port=6
  Vod : Outport  Port=7
  Vod_s : Outport  Port=8
  wo_s : Outport  Port=9
  wires:
  Gain/1 -> dq converter/2(Iodq)
  Droop for secondary control2/2(wt) -> [wt], dq converter/4(wo), 3to2 3/2("wt ")
  Gain2/1 -> Low-pass filter/2(q_hat)
  PQ calculator/2(q_hat) -> Gain2/1
  Gain1/1 -> Low-pass filter/1(p_hat)
  dq converter/2(Voq) -> PQ calculator/2(Voq)
  PQ calculator/1(p_hat) -> Scope1/1, Gain1/1
  dq converter/1(Vod) -> Vod/1, PQ calculator/1(Vod)
  [Vo] -> Selector2/1, Vo/1
  [Io] -> Io/1
  Three-Phase V-I Measurement/1 -> [Vo]
  Three-Phase V-I Measurement/2 -> [Io]
  Three-Phase V-I Measurement1/2 -> [Il]
  3to2 1/1(Vo) -> "Model Predictive Control "/1(Vc)
  3to2 3/1(threePhase) -> "Model Predictive Control "/3(vref)  "vref"
  3to2 2/1(Il) -> "Model Predictive Control "/2(i_filter)
  "Model Predictive Control "/2(Sopt) -> remap/1(In1)
  Gain3/1 -> dq converter/3(Ildq), 3to2 2/1("Iabc_o ")
  remap/1(Out1) -> Two-Level Converter/1
  [Vo] -> Zero-Order Hold/1
  [Io] -> Zero-Order Hold1/1
  [Il] -> Zero-Order Hold2/1
  Droop for secondary control2/1(Vref) -> 3to2 3/1("single ")
  Three-Phase V-I Measurement1/1 -> Demux/1
  Demux/1 -> Counter/1, Scope5/2  "Input Signal"
  Clock/1 -> Divide/2
  Reset every 1 second/1 -> Scope5/1, Counter/2  "Reset Intervals(secs)"
  Counter/1 -> Scope5/3, Divide/1  "Counts"
  Divide/1 -> Scope5/4  "Frequency"
  dq converter/4(Ioq) -> PQ calculator/4(Ioq)
  Low-pass filter/2(Q) -> Droop for secondary control2/4(Q), Q/1  "Q"
  dq converter/3(Iod) -> PQ calculator/3(Iod)
  Droop for secondary control2/3(wo) -> wo1/1
  Low-pass filter/1(P) -> Scope2/1, Droop for secondary control2/1(P), P/1  "P"
  Sum1/1 -> Droop for secondary control2/2(w_nom)
  V_nom1/1 -> Droop for secondary control2/3(V_nom)
  CDSC-PLL/2(Vd) -> Vod_s/1
  Low-Pass Filter (Discrete or Continuous)/1 -> Gain5/1
  Gain5/1 -> theta/1
  Product1/1 -> Low-Pass Filter (Discrete or Continuous)/1
  Selector2/1 -> Product1/1
  Selector3/1 -> Product1/2
  [delay] -> Switch2/2
  Switch2/1 -> Sum1/1
  w_nom2/1 -> Switch2/3
  w_nom1/1 -> Sum1/2
  wni/1 -> Switch2/1
  Zero-Order Hold/1 -> dq converter/1(Vodq), 3to2 1/1("Vabc_o ")
  Zero-Order Hold1/1 -> Gain/1
  Zero-Order Hold2/1 -> Gain3/1
  Bus 1/1 -> CDSC-PLL/1(abc), Selector3/1
  CDSC-PLL/1(w) -> wo_s/1
  connections:
  Three-Phase Series RLC Branch2/LConn1 -- Three-Phase V-I Measurement/RConn1 -- Three-Phase Series RLC Branch/LConn1
  Two-Level Converter/RConn1 -- DC Voltage Source1/RConn1 -- Series RLC Branch/LConn1
  Three-Phase Series RLC Branch2/RConn3 -- Three-Phase Series RLC Branch2/RConn1 -- Three-Phase Series RLC Branch2/RConn2
  Three-Phase Series RLC Branch2/LConn3 -- Three-Phase Series RLC Branch/LConn3 -- Three-Phase V-I Measurement/RConn3
  Two-Level Converter/RConn2 -- Series RLC Branch/RConn1 -- DC Voltage Source1/LConn1
  Three-Phase Series RLC Branch/LConn2 -- Three-Phase V-I Measurement/RConn2 -- Three-Phase Series RLC Branch2/LConn2
  Two-Level Converter/LConn1 -- Three-Phase V-I Measurement1/RConn1
  Three-Phase V-I Measurement1/LConn2 -- Three-Phase Series RLC Branch/RConn2
  Two-Level Converter/LConn2 -- Three-Phase V-I Measurement1/RConn2
  Two-Level Converter/LConn3 -- Three-Phase V-I Measurement1/RConn3
  Three-Phase Series RLC Branch/RConn1 -- Three-Phase V-I Measurement1/LConn1
  Three-Phase V-I Measurement/LConn1 -- Three-Phase Series RLC Branch1/RConn1
  Three-Phase V-I Measurement/LConn2 -- Three-Phase Series RLC Branch1/RConn2
  Three-Phase Series RLC Branch1/RConn3 -- Three-Phase V-I Measurement/LConn3
  Three-Phase Series RLC Branch/RConn3 -- Three-Phase V-I Measurement1/LConn3
  Conn1/RConn1 -- Bus 1/LConn1
  Conn2/RConn1 -- Bus 1/LConn2
  Conn3/RConn1 -- Bus 1/LConn3
  Bus 1/RConn1 -- Three-Phase Series RLC Branch1/LConn1
  Bus 1/RConn2 -- Three-Phase Series RLC Branch1/LConn2
  Bus 1/RConn3 -- Three-Phase Series RLC Branch1/LConn3
